simulink model "case9"  (R2024b)
settings: Solver=FixedStepAuto  StartTime=0  StopTime=1  FixedStep=1e-7  RelTol=1e-3
values from neighbouring files (symbols this model uses):
  SG_D_1_D = 0.01056    [IEEE9_case_parameters.m]    (also in case1_parameters.m; case2_parameters.m; case3_parameters.m; case4_parameters.m)
  SG_D_1_EnableSaturation = 0    [IEEE9_case_parameters.m]    (also in case1_parameters.m; case2_parameters.m; case3_parameters.m; case4_parameters.m)
  SG_D_1_f0 = 60    [IEEE9_case_parameters.m]    (also in case1_parameters.m; case2_parameters.m; case3_parameters.m; case4_parameters.m)
  SG_D_1_H = 7.5    [IEEE9_case_parameters.m]    (also in case1_parameters.m; case2_parameters.m; case3_parameters.m; case4_parameters.m)
  SG_D_1_K_A = 20    [IEEE9_case_parameters.m]    (also in case1_parameters.m; case2_parameters.m; case3_parameters.m; case4_parameters.m)
  SG_D_1_K_E = 1.000000e+1    (= 10)    [IEEE9_case_parameters.m]    (also in case1_parameters.m; case2_parameters.m; case3_parameters.m; case4_parameters.m)
  SG_D_1_K_F = 2.363    [IEEE9_case_parameters.m]    (also in case1_parameters.m; case2_parameters.m; case3_parameters.m; case4_parameters.m)
  SG_D_1_K_s = 0.5    [IEEE9_case_parameters.m]    (also in case1_parameters.m = 5; case2_parameters.m = 5; case3_parameters.m = 5; case4_parameters.m = 5)
  SG_D_1_R_a = 0.001088    [IEEE9_case_parameters.m]    (also in case1_parameters.m; case2_parameters.m; case3_parameters.m; case4_parameters.m)
  SG_D_1_S_A = 1    [IEEE9_case_parameters.m]    (also in case1_parameters.m; case2_parameters.m; case3_parameters.m; case4_parameters.m)
  SG_D_1_S_B = 0.103    [IEEE9_case_parameters.m]    (also in case1_parameters.m; case2_parameters.m; case3_parameters.m; case4_parameters.m)
  SG_D_1_S_N = 10.659857    [IEEE9_case_parameters.m]    (also in case1_parameters.m; case2_parameters.m; case3_parameters.m; case4_parameters.m)
  SG_D_1_SpeedPara = 200    [IEEE9_case_parameters.m]    (also in case1_parameters.m; case2_parameters.m; case3_parameters.m; case4_parameters.m)
  SG_D_1_T_0 = 0.720173    [IEEE9_case_parameters.m]    (also in case1_parameters.m = 0.755522; case2_parameters.m = 0.808931; case3_parameters.m = 0.869402; case4_parameters.m = 0.729316)
  SG_D_1_T_1 = 0.3    [IEEE9_case_parameters.m]    (also in case1_parameters.m; case2_parameters.m; case3_parameters.m; case4_parameters.m)
  SG_D_1_T_2 = 0.05    [IEEE9_case_parameters.m]    (also in case1_parameters.m; case2_parameters.m; case3_parameters.m; case4_parameters.m)
  SG_D_1_T_3 = 0.02    [IEEE9_case_parameters.m]    (also in case1_parameters.m; case2_parameters.m; case3_parameters.m; case4_parameters.m)
  SG_D_1_T_4 = 0.005    [IEEE9_case_parameters.m]    (also in case1_parameters.m; case2_parameters.m; case3_parameters.m; case4_parameters.m)
  SG_D_1_T_A = 0.02    [IEEE9_case_parameters.m]    (also in case1_parameters.m; case2_parameters.m; case3_parameters.m; case4_parameters.m)
  SG_D_1_T_dd = 8.000000e+0    (= 8)    [IEEE9_case_parameters.m]    (also in case1_parameters.m; case2_parameters.m; case3_parameters.m; case4_parameters.m)
  SG_D_1_T_ddd = 0.04    [IEEE9_case_parameters.m]    (also in case1_parameters.m; case2_parameters.m; case3_parameters.m; case4_parameters.m)
  SG_D_1_T_E = 0.314    [IEEE9_case_parameters.m]    (also in case1_parameters.m; case2_parameters.m; case3_parameters.m; case4_parameters.m)
  SG_D_1_T_F = 0.35    [IEEE9_case_parameters.m]    (also in case1_parameters.m; case2_parameters.m; case3_parameters.m; case4_parameters.m)
  SG_D_1_T_qd = 0.8    [IEEE9_case_parameters.m]    (also in case1_parameters.m; case2_parameters.m; case3_parameters.m; case4_parameters.m)
  SG_D_1_T_qdd = 0.02    [IEEE9_case_parameters.m]    (also in case1_parameters.m; case2_parameters.m; case3_parameters.m; case4_parameters.m)
  SG_D_1_T_speed = 0.1    [IEEE9_case_parameters.m]    (also in case1_parameters.m = 200; case2_parameters.m = 200; case3_parameters.m = 200; case4_parameters.m = 200)
  SG_D_1_T_w = 0.5    [IEEE9_case_parameters.m]    (also in case1_parameters.m; case2_parameters.m; case3_parameters.m; case4_parameters.m)
  SG_D_1_V_ref = 1.990276    [IEEE9_case_parameters.m]    (also in case1_parameters.m = 2.042296; case2_parameters.m = 2.051388; case3_parameters.m = 2.089584; case4_parameters.m = 2.01845)
  SG_D_1_w_ref = 376.991118    [IEEE9_case_parameters.m]    (also in case1_parameters.m; case2_parameters.m; case3_parameters.m; case4_parameters.m)
  SG_D_1_wb = 6.000000e+1    (= 60)    [IEEE9_case_parameters.m]    (also in case1_parameters.m; case2_parameters.m; case3_parameters.m; case4_parameters.m)
  SG_D_1_x_d = 1.9    [IEEE9_case_parameters.m]    (also in case1_parameters.m; case2_parameters.m; case3_parameters.m; case4_parameters.m)
  SG_D_1_x_dd = 0.302    [IEEE9_case_parameters.m]    (also in case1_parameters.m; case2_parameters.m; case3_parameters.m; case4_parameters.m)
  SG_D_1_x_ddd = 0.204    [IEEE9_case_parameters.m]    (also in case1_parameters.m; case2_parameters.m; case3_parameters.m; case4_parameters.m)
  SG_D_1_x_l = 0.05    [IEEE9_case_parameters.m]    (also in case1_parameters.m; case2_parameters.m; case3_parameters.m; case4_parameters.m)
  SG_D_1_x_q = 1.3    [IEEE9_case_parameters.m]    (also in case1_parameters.m; case2_parameters.m; case3_parameters.m; case4_parameters.m)
  SG_D_1_x_qd = 0.5    [IEEE9_case_parameters.m]    (also in case1_parameters.m; case2_parameters.m; case3_parameters.m; case4_parameters.m)
  SG_D_1_x_qdd = 0.3    [IEEE9_case_parameters.m]    (also in case1_parameters.m; case2_parameters.m; case3_parameters.m; case4_parameters.m)
  SG_D_2_D = 0.02    [IEEE9_case_parameters.m]    (also in case1_parameters.m; case2_parameters.m; case3_parameters.m; case4_parameters.m)
  SG_D_2_EnableSaturation = 0    [IEEE9_case_parameters.m]    (also in case1_parameters.m; case2_parameters.m; case3_parameters.m; case4_parameters.m)
  SG_D_2_f0 = 60    [IEEE9_case_parameters.m]    (also in case1_parameters.m; case2_parameters.m; case3_parameters.m; case4_parameters.m)
  SG_D_2_H = 8.000000e+0    (= 8)    [IEEE9_case_parameters.m]    (also in case1_parameters.m; case2_parameters.m; case3_parameters.m; case4_parameters.m)
  SG_D_2_K_A = 20    [IEEE9_case_parameters.m]    (also in case1_parameters.m; case2_parameters.m; case3_parameters.m; case4_parameters.m)
  SG_D_2_K_E = 1.000000e+1    (= 10)    [IEEE9_case_parameters.m]    (also in case1_parameters.m; case2_parameters.m; case3_parameters.m; case4_parameters.m)
  SG_D_2_K_F = 2.363    [IEEE9_case_parameters.m]    (also in case1_parameters.m; case2_parameters.m; case3_parameters.m; case4_parameters.m)
  SG_D_2_K_s = 0.5    [IEEE9_case_parameters.m]    (also in case1_parameters.m = 4; case2_parameters.m = 4; case3_parameters.m = 4; case4_parameters.m = 4)
  SG_D_2_R_a = 0.001088    [IEEE9_case_parameters.m]    (also in case1_parameters.m; case2_parameters.m; case3_parameters.m; case4_parameters.m)
  SG_D_2_S_A = 1    [IEEE9_case_parameters.m]    (also in case1_parameters.m; case2_parameters.m; case3_parameters.m; case4_parameters.m)
  SG_D_2_S_B = 0.103    [IEEE9_case_parameters.m]    (also in case1_parameters.m; case2_parameters.m; case3_parameters.m; case4_parameters.m)
  SG_D_2_S_N = 10.659857    [IEEE9_case_parameters.m]    (also in case1_parameters.m; case2_parameters.m; case3_parameters.m; case4_parameters.m)
  SG_D_2_SpeedPara = 200    [IEEE9_case_parameters.m]    (also in case1_parameters.m; case2_parameters.m; case3_parameters.m; case4_parameters.m)
  SG_D_2_T_0 = 1.632913    [IEEE9_case_parameters.m]    (also in case1_parameters.m = 1.632925; case2_parameters.m = 1.632915; case3_parameters.m = 1.632914; case4_parameters.m = 1.632927)
  SG_D_2_T_1 = 0.2    [IEEE9_case_parameters.m]    (also in case1_parameters.m; case2_parameters.m; case3_parameters.m; case4_parameters.m)
  SG_D_2_T_2 = 0.05    [IEEE9_case_parameters.m]    (also in case1_parameters.m; case2_parameters.m; case3_parameters.m; case4_parameters.m)
  SG_D_2_T_3 = 0.02    [IEEE9_case_parameters.m]    (also in case1_parameters.m; case2_parameters.m; case3_parameters.m; case4_parameters.m)
  SG_D_2_T_4 = 0.005    [IEEE9_case_parameters.m]    (also in case1_parameters.m; case2_parameters.m; case3_parameters.m; case4_parameters.m)
  SG_D_2_T_A = 0.02    [IEEE9_case_parameters.m]    (also in case1_parameters.m; case2_parameters.m; case3_parameters.m; case4_parameters.m)
  SG_D_2_T_dd = 7.9    [IEEE9_case_parameters.m]    (also in case1_parameters.m; case2_parameters.m; case3_parameters.m; case4_parameters.m)
  SG_D_2_T_ddd = 0.04    [IEEE9_case_parameters.m]    (also in case1_parameters.m; case2_parameters.m; case3_parameters.m; case4_parameters.m)
  SG_D_2_T_E = 0.314    [IEEE9_case_parameters.m]    (also in case1_parameters.m; case2_parameters.m; case3_parameters.m; case4_parameters.m)
  SG_D_2_T_F = 0.35    [IEEE9_case_parameters.m]    (also in case1_parameters.m; case2_parameters.m; case3_parameters.m; case4_parameters.m)
  SG_D_2_T_qd = 0.8    [IEEE9_case_parameters.m]    (also in case1_parameters.m; case2_parameters.m; case3_parameters.m; case4_parameters.m)
  SG_D_2_T_qdd = 0.015    [IEEE9_case_parameters.m]    (also in case1_parameters.m; case2_parameters.m; case3_parameters.m; case4_parameters.m)
  SG_D_2_T_speed = 0.1    [IEEE9_case_parameters.m]    (also in case1_parameters.m = 150; case2_parameters.m = 150; case3_parameters.m = 150; case4_parameters.m = 150)
  SG_D_2_T_w = 0.35    [IEEE9_case_parameters.m]    (also in case1_parameters.m; case2_parameters.m; case3_parameters.m; case4_parameters.m)
  SG_D_2_V_ref = 2.58547    [IEEE9_case_parameters.m]    (also in case1_parameters.m = 2.597896; case2_parameters.m = 2.587136; case3_parameters.m = 2.586042; case4_parameters.m = 2.599679)
  SG_D_2_w_ref = 376.991118    [IEEE9_case_parameters.m]    (also in case1_parameters.m; case2_parameters.m; case3_parameters.m; case4_parameters.m)
  SG_D_2_wb = 6.000000e+1    (= 60)    [IEEE9_case_parameters.m]    (also in case1_parameters.m; case2_parameters.m; case3_parameters.m; case4_parameters.m)
  SG_D_2_x_d = 1.8    [IEEE9_case_parameters.m]    (also in case1_parameters.m; case2_parameters.m; case3_parameters.m; case4_parameters.m)
  SG_D_2_x_dd = 0.302    [IEEE9_case_parameters.m]    (also in case1_parameters.m; case2_parameters.m; case3_parameters.m; case4_parameters.m)
  SG_D_2_x_ddd = 0.204    [IEEE9_case_parameters.m]    (also in case1_parameters.m; case2_parameters.m; case3_parameters.m; case4_parameters.m)
  SG_D_2_x_l = 0.05    [IEEE9_case_parameters.m]    (also in case1_parameters.m; case2_parameters.m; case3_parameters.m; case4_parameters.m)
  SG_D_2_x_q = 1.25    [IEEE9_case_parameters.m]    (also in case1_parameters.m; case2_parameters.m; case3_parameters.m; case4_parameters.m)
  SG_D_2_x_qd = 0.5    [IEEE9_case_parameters.m]    (also in case1_parameters.m; case2_parameters.m; case3_parameters.m; case4_parameters.m)
  SG_D_2_x_qdd = 0.3    [IEEE9_case_parameters.m]    (also in case1_parameters.m; case2_parameters.m; case3_parameters.m; case4_parameters.m)
  SG_D_3_D = 0.02    [IEEE9_case_parameters.m]    (also in case1_parameters.m; case2_parameters.m; case3_parameters.m; case4_parameters.m)
  SG_D_3_EnableSaturation = 0    [IEEE9_case_parameters.m]    (also in case1_parameters.m; case2_parameters.m; case3_parameters.m; case4_parameters.m)
  SG_D_3_f0 = 60    [IEEE9_case_parameters.m]    (also in case1_parameters.m; case2_parameters.m; case3_parameters.m; case4_parameters.m)
  SG_D_3_H = 7.7    [IEEE9_case_parameters.m]    (also in case1_parameters.m; case2_parameters.m; case3_parameters.m; case4_parameters.m)
  SG_D_3_K_A = 20    [IEEE9_case_parameters.m]    (also in case1_parameters.m; case2_parameters.m; case3_parameters.m; case4_parameters.m)
  SG_D_3_K_E = 1.000000e+1    (= 10)    [IEEE9_case_parameters.m]    (also in case1_parameters.m; case2_parameters.m; case3_parameters.m; case4_parameters.m)
  SG_D_3_K_F = 2.363    [IEEE9_case_parameters.m]    (also in case1_parameters.m; case2_parameters.m; case3_parameters.m; case4_parameters.m)
  SG_D_3_K_s = 0.2    [IEEE9_case_parameters.m]    (also in case1_parameters.m = 2; case2_parameters.m = 2; case3_parameters.m = 2; case4_parameters.m = 2)
  SG_D_3_R_a = 0.001088    [IEEE9_case_parameters.m]    (also in case1_parameters.m; case2_parameters.m; case3_parameters.m; case4_parameters.m)
  SG_D_3_S_A = 1    [IEEE9_case_parameters.m]    (also in case1_parameters.m; case2_parameters.m; case3_parameters.m; case4_parameters.m)
  SG_D_3_S_B = 0.103    [IEEE9_case_parameters.m]    (also in case1_parameters.m; case2_parameters.m; case3_parameters.m; case4_parameters.m)
  SG_D_3_S_N = 10.659857    [IEEE9_case_parameters.m]    (also in case1_parameters.m; case2_parameters.m; case3_parameters.m; case4_parameters.m)
  SG_D_3_SpeedPara = 200    [IEEE9_case_parameters.m]    (also in case1_parameters.m; case2_parameters.m; case3_parameters.m; case4_parameters.m)
  SG_D_3_T_0 = 0.850788    [IEEE9_case_parameters.m]    (also in case1_parameters.m = 0.850786; case2_parameters.m = 0.850787; case3_parameters.m; case4_parameters.m = 0.850786)
  SG_D_3_T_1 = 0.2    [IEEE9_case_parameters.m]    (also in case1_parameters.m; case2_parameters.m; case3_parameters.m; case4_parameters.m)
  SG_D_3_T_2 = 0.05    [IEEE9_case_parameters.m]    (also in case1_parameters.m; case2_parameters.m; case3_parameters.m; case4_parameters.m)
  SG_D_3_T_3 = 0.02    [IEEE9_case_parameters.m]    (also in case1_parameters.m; case2_parameters.m; case3_parameters.m; case4_parameters.m)
  SG_D_3_T_4 = 0.005    [IEEE9_case_parameters.m]    (also in case1_parameters.m; case2_parameters.m; case3_parameters.m; case4_parameters.m)
  SG_D_3_T_A = 0.02    [IEEE9_case_parameters.m]    (also in case1_parameters.m; case2_parameters.m; case3_parameters.m; case4_parameters.m)
  SG_D_3_T_dd = 8.1    [IEEE9_case_parameters.m]    (also in case1_parameters.m; case2_parameters.m; case3_parameters.m; case4_parameters.m)
  SG_D_3_T_ddd = 0.04    [IEEE9_case_parameters.m]    (also in case1_parameters.m; case2_parameters.m; case3_parameters.m; case4_parameters.m)
  SG_D_3_T_E = 0.314    [IEEE9_case_parameters.m]    (also in case1_parameters.m; case2_parameters.m; case3_parameters.m; case4_parameters.m)
  SG_D_3_T_F = 0.35    [IEEE9_case_parameters.m]    (also in case1_parameters.m; case2_parameters.m; case3_parameters.m; case4_parameters.m)
  SG_D_3_T_qd = 0.8    [IEEE9_case_parameters.m]    (also in case1_parameters.m; case2_parameters.m; case3_parameters.m; case4_parameters.m)
  SG_D_3_T_qdd = 0.015    [IEEE9_case_parameters.m]    (also in case1_parameters.m; case2_parameters.m; case3_parameters.m; case4_parameters.m)
  SG_D_3_T_speed = 0.1    [IEEE9_case_parameters.m]    (also in case1_parameters.m = 180; case2_parameters.m = 180; case3_parameters.m = 180; case4_parameters.m = 180)
  SG_D_3_T_w = 0.4    [IEEE9_case_parameters.m]    (also in case1_parameters.m; case2_parameters.m; case3_parameters.m; case4_parameters.m)
  SG_D_3_V_ref = 1.892727    [IEEE9_case_parameters.m]    (also in case1_parameters.m = 1.906439; case2_parameters.m = 1.895535; case3_parameters.m = 1.892105; case4_parameters.m = 1.906598)
  SG_D_3_w_ref = 376.991118    [IEEE9_case_parameters.m]    (also in case1_parameters.m; case2_parameters.m; case3_parameters.m; case4_parameters.m)
  SG_D_3_wb = 6.000000e+1    (= 60)    [IEEE9_case_parameters.m]    (also in case1_parameters.m; case2_parameters.m; case3_parameters.m; case4_parameters.m)
  SG_D_3_x_d = 1.85    [IEEE9_case_parameters.m]    (also in case1_parameters.m; case2_parameters.m; case3_parameters.m; case4_parameters.m)
  SG_D_3_x_dd = 0.302    [IEEE9_case_parameters.m]    (also in case1_parameters.m; case2_parameters.m; case3_parameters.m; case4_parameters.m)
  SG_D_3_x_ddd = 0.204    [IEEE9_case_parameters.m]    (also in case1_parameters.m; case2_parameters.m; case3_parameters.m; case4_parameters.m)
  SG_D_3_x_l = 0.05    [IEEE9_case_parameters.m]    (also in case1_parameters.m; case2_parameters.m; case3_parameters.m; case4_parameters.m)
  SG_D_3_x_q = 1.2    [IEEE9_case_parameters.m]    (also in case1_parameters.m; case2_parameters.m; case3_parameters.m; case4_parameters.m)
  SG_D_3_x_qd = 0.5    [IEEE9_case_parameters.m]    (also in case1_parameters.m; case2_parameters.m; case3_parameters.m; case4_parameters.m)
  SG_D_3_x_qdd = 0.3    [IEEE9_case_parameters.m]    (also in case1_parameters.m; case2_parameters.m; case3_parameters.m; case4_parameters.m)
(part 2 of 12)

== system case9/AC_1/d_id_line_8_9_block ==
  note: d_id_line_8_9 in case9
      | $376.991118430775\,\mathrm{iq}_{\mathrm{line},8,9}-79.079547273782\,\mathrm{id}_{\mathrm{line},8,9}+2308.03849601368\,\mathrm{vd}_{\mathrm{bus},8}-2308.03849601368\,\mathrm{vd}_{\mathrm{bus},9}$
      | Automatically generated on 2025-10-31 19:35:46 .
  State_id_line_8_9_7f57b : Inport
  State_iq_line_8_9_a0851 : Inport  Port=2
  State_vd_bus_8_2850b : Inport  Port=3
  State_vd_bus_9_05d0b : Inport  Port=4
  Add_7d5a3 : Sum
  Add_dee88 : Sum
  Constant_-79.079547273782_7223d : Constant  Value=-79.079547273782
  Constant_2308.03849601368_486f2 : Constant  Value=2308.03849601368
  Constant_2308.03849601368_a27ee : Constant  Value=2308.03849601368
  Constant_376.991118430775_3d7fd : Constant  Value=376.991118430775
  Product_07161 : Product
  Product_cf3c9 : Product
  Product_d47ae : Product
  Product_f756a : Product
  Subtract_736c3 : Sum  Inputs=+-
  Blockout_d_id_line_8_9_34a3f : Outport
  wires:
  Constant_-79.079547273782_7223d/1 -> Product_d47ae/1
  Product_f756a/1 -> Add_7d5a3/2
  State_id_line_8_9_7f57b/1 -> Product_d47ae/2
  Constant_376.991118430775_3d7fd/1 -> Product_f756a/1
  State_iq_line_8_9_a0851/1 -> Product_f756a/2
  Product_d47ae/1 -> Add_7d5a3/1
  Constant_2308.03849601368_486f2/1 -> Product_07161/1
  State_vd_bus_8_2850b/1 -> Product_07161/2
  Add_7d5a3/1 -> Add_dee88/1
  Product_07161/1 -> Add_dee88/2
  Constant_2308.03849601368_a27ee/1 -> Product_cf3c9/1
  State_vd_bus_9_05d0b/1 -> Product_cf3c9/2
  Add_dee88/1 -> Subtract_736c3/1
  Product_cf3c9/1 -> Subtract_736c3/2
  Subtract_736c3/1 -> Blockout_d_id_line_8_9_34a3f/1

== system case9/AC_1/d_id_line_9_4_block ==
  note: d_id_line_9_4 in case9
      | $376.991118430775\,\mathrm{iq}_{\mathrm{line},9,4}-46.8081143789666\,\mathrm{id}_{\mathrm{line},9,4}-4371.69644539061\,\mathrm{vd}_{\mathrm{bus},4}+4371.69644539061\,\mathrm{vd}_{\mathrm{bus},9}$
      | Automatically generated on 2025-10-31 19:35:47 .
  State_id_line_9_4_2f88c : Inport
  State_iq_line_9_4_5e3d8 : Inport  Port=2
  State_vd_bus_4_6d2a8 : Inport  Port=3
  State_vd_bus_9_2d37e : Inport  Port=4
  Add_5ea3d : Sum
  Add_7fd3a : Sum
  Constant_-46.8081143789666_5ee22 : Constant  Value=-46.8081143789666
  Constant_376.991118430775_a2f3b : Constant  Value=376.991118430775
  Constant_4371.69644539061_67045 : Constant  Value=4371.69644539061
  Constant_4371.69644539061_93ce0 : Constant  Value=4371.69644539061
  Product_23b32 : Product
  Product_5d2fa : Product
  Product_c4883 : Product
  Product_f07a4 : Product
  Subtract_26f71 : Sum  Inputs=+-
  Blockout_d_id_line_9_4_009d8 : Outport
  wires:
  Constant_-46.8081143789666_5ee22/1 -> Product_c4883/1
  Product_23b32/1 -> Add_5ea3d/2
  State_id_line_9_4_2f88c/1 -> Product_c4883/2
  Constant_376.991118430775_a2f3b/1 -> Product_23b32/1
  Product_c4883/1 -> Add_5ea3d/1
  State_iq_line_9_4_5e3d8/1 -> Product_23b32/2
  Constant_4371.69644539061_67045/1 -> Product_f07a4/1
  State_vd_bus_4_6d2a8/1 -> Product_f07a4/2
  Add_5ea3d/1 -> Subtract_26f71/1
  Product_f07a4/1 -> Subtract_26f71/2
  Constant_4371.69644539061_93ce0/1 -> Product_5d2fa/1
  Subtract_26f71/1 -> Add_7fd3a/1
  State_vd_bus_9_2d37e/1 -> Product_5d2fa/2
  Product_5d2fa/1 -> Add_7fd3a/2
  Add_7fd3a/1 -> Blockout_d_id_line_9_4_009d8/1

== system case9/AC_1/d_id_load_5_block ==
  note: d_id_load_5 in case9
      | $376.991118430775\,\mathrm{iq}_{\mathrm{load},5}-1271.35173163011\,\mathrm{id}_{\mathrm{load},5}+1369.24920855552\,\mathrm{vd}_{\mathrm{bus},5}$
      | Automatically generated on 2025-10-31 19:35:37 .
  State_id_load_5_0cf96 : Inport
  State_iq_load_5_0d2e0 : Inport  Port=2
  State_vd_bus_5_6d5a2 : Inport  Port=3
  Add_3aace : Sum
  Add_6ece1 : Sum
  Constant_-1271.35173163011_4a864 : Constant  Value=-1271.35173163011
  Constant_1369.24920855552_9b5a8 : Constant  Value=1369.24920855552
  Constant_376.991118430775_69578 : Constant  Value=376.991118430775
  Product_78272 : Product
  Product_da222 : Product
  Product_dfef5 : Product
  Blockout_d_id_load_5_39313 : Outport
  wires:
  Constant_-1271.35173163011_4a864/1 -> Product_78272/1
  Product_dfef5/1 -> Add_6ece1/2
  State_id_load_5_0cf96/1 -> Product_78272/2
  Constant_376.991118430775_69578/1 -> Product_dfef5/1
  Product_da222/1 -> Add_3aace/2
  State_iq_load_5_0d2e0/1 -> Product_dfef5/2
  Product_78272/1 -> Add_6ece1/1
  Constant_1369.24920855552_9b5a8/1 -> Product_da222/1
  State_vd_bus_5_6d5a2/1 -> Product_da222/2
  Add_6ece1/1 -> Add_3aace/1
  Add_3aace/1 -> Blockout_d_id_load_5_39313/1

== system case9/AC_1/d_id_load_7_block ==
  note: d_id_load_7 in case9
      | $376.991118430775\,\mathrm{iq}_{\mathrm{load},7}-1210.81117316871\,\mathrm{id}_{\mathrm{load},7}+1430.28886940914\,\mathrm{vd}_{\mathrm{bus},7}$
      | Automatically generated on 2025-10-31 19:35:38 .
  State_id_load_7_475ab : Inport
  State_iq_load_7_faf72 : Inport  Port=2
  State_vd_bus_7_54001 : Inport  Port=3
  Add_78a86 : Sum
  Add_d7d34 : Sum
  Constant_-1210.81117316871_adc5d : Constant  Value=-1210.81117316871
  Constant_1430.28886940914_d6361 : Constant  Value=1430.28886940914
  Constant_376.991118430775_fd455 : Constant  Value=376.991118430775
  Product_c0859 : Product
  Product_ea5b8 : Product
  Product_fa99e : Product
  Blockout_d_id_load_7_24cac : Outport
  wires:
  Constant_-1210.81117316871_adc5d/1 -> Product_fa99e/1
  Product_c0859/1 -> Add_78a86/2
  State_id_load_7_475ab/1 -> Product_fa99e/2
  Constant_376.991118430775_fd455/1 -> Product_c0859/1
  Product_fa99e/1 -> Add_78a86/1
  State_iq_load_7_faf72/1 -> Product_c0859/2
  Constant_1430.28886940914_d6361/1 -> Product_ea5b8/1
  State_vd_bus_7_54001/1 -> Product_ea5b8/2
  Add_78a86/1 -> Add_d7d34/1
  Product_ea5b8/1 -> Add_d7d34/2
  Add_d7d34/1 -> Blockout_d_id_load_7_24cac/1

== system case9/AC_1/d_id_load_9_block ==
  note: d_id_load_9 in case9
      | $376.991118430775\,\mathrm{iq}_{\mathrm{load},9}-1059.45977647\,\mathrm{id}_{\mathrm{load},9}+1700.21710984812\,\mathrm{vd}_{\mathrm{bus},9}$
      | Automatically generated on 2025-10-31 19:35:39 .
  State_id_load_9_9c654 : Inport
  State_iq_load_9_9f0e2 : Inport  Port=2
  State_vd_bus_9_61c11 : Inport  Port=3
  Add_3c334 : Sum
  Add_4cb1c : Sum
  Constant_-1059.45977647_80d06 : Constant  Value=-1059.45977647
  Constant_1700.21710984812_ffb11 : Constant  Value=1700.21710984812
  Constant_376.991118430775_49f56 : Constant  Value=376.991118430775
  Product_15e95 : Product
  Product_2c0b1 : Product
  Product_f7556 : Product
  Blockout_d_id_load_9_7efdf : Outport
  wires:
  Constant_-1059.45977647_80d06/1 -> Product_15e95/1
  Product_2c0b1/1 -> Add_3c334/2
  State_id_load_9_9c654/1 -> Product_15e95/2
  Constant_376.991118430775_49f56/1 -> Product_2c0b1/1
  Product_15e95/1 -> Add_3c334/1
  State_iq_load_9_9f0e2/1 -> Product_2c0b1/2
  Constant_1700.21710984812_ffb11/1 -> Product_f7556/1
  State_vd_bus_9_61c11/1 -> Product_f7556/2
  Add_3c334/1 -> Add_4cb1c/1
  Product_f7556/1 -> Add_4cb1c/2
  Add_4cb1c/1 -> Blockout_d_id_load_9_7efdf/1

== system case9/AC_1/d_iq_line_1_4_block ==
  note: d_iq_line_1_4 in case9
      | $6451.28815726045\,\mathrm{vq}_{\mathrm{bus},1}-376.991118430775\,\mathrm{id}_{\mathrm{line},1,4}-6451.28815726045\,\mathrm{vq}_{\mathrm{bus},4}$
      | Automatically generated on 2025-10-31 19:35:40 .
  State_id_line_1_4_4a24e : Inport
  State_vq_bus_1_3337a : Inport  Port=2
  State_vq_bus_4_a6b34 : Inport  Port=3
  Add_6db9b : Sum
  Constant_-376.991118430775_70d78 : Constant  Value=-376.991118430775
  Constant_6451.28815726045_2aa38 : Constant  Value=6451.28815726045
  Constant_6451.28815726045_82ff4 : Constant  Value=6451.28815726045
  Product_6c42f : Product
  Product_b527a : Product
  Product_fcdd1 : Product
  Subtract_113de : Sum  Inputs=+-
  Blockout_d_iq_line_1_4_3376e : Outport
  wires:
  Constant_-376.991118430775_70d78/1 -> Product_b527a/1
  Product_fcdd1/1 -> Add_6db9b/2
  State_id_line_1_4_4a24e/1 -> Product_b527a/2
  Constant_6451.28815726045_82ff4/1 -> Product_fcdd1/1
  Product_b527a/1 -> Add_6db9b/1
  Subtract_113de/1 -> Blockout_d_iq_line_1_4_3376e/1
  State_vq_bus_1_3337a/1 -> Product_fcdd1/2
  Constant_6451.28815726045_2aa38/1 -> Product_6c42f/1
  State_vq_bus_4_a6b34/1 -> Product_6c42f/2
  Add_6db9b/1 -> Subtract_113de/1
  Product_6c42f/1 -> Subtract_113de/2

== system case9/AC_1/d_iq_line_3_6_block ==
  note: d_iq_line_3_6 in case9
      | $6341.19791566897\,\mathrm{vq}_{\mathrm{bus},3}-376.991118430775\,\mathrm{id}_{\mathrm{line},3,6}-6341.19791566897\,\mathrm{vq}_{\mathrm{bus},6}$
      | Automatically generated on 2025-10-31 19:35:43 .
  State_id_line_3_6_aaf98 : Inport
  State_vq_bus_3_d110b : Inport  Port=2
  State_vq_bus_6_cc5e9 : Inport  Port=3
  Add_271bd : Sum
  Constant_-376.991118430775_89aa7 : Constant  Value=-376.991118430775
  Constant_6341.19791566897_20e3c : Constant  Value=6341.19791566897
  Constant_6341.19791566897_be9af : Constant  Value=6341.19791566897
  Product_900cb : Product
  Product_e38f3 : Product
  Product_e9343 : Product
  Subtract_02134 : Sum  Inputs=+-
  Blockout_d_iq_line_3_6_fff78 : Outport
  wires:
  Constant_-376.991118430775_89aa7/1 -> Product_e38f3/1
  Product_e9343/1 -> Add_271bd/2
  State_id_line_3_6_aaf98/1 -> Product_e38f3/2
  Constant_6341.19791566897_20e3c/1 -> Product_e9343/1
  Product_e38f3/1 -> Add_271bd/1
  State_vq_bus_3_d110b/1 -> Product_e9343/2
  Constant_6341.19791566897_be9af/1 -> Product_900cb/1
  State_vq_bus_6_cc5e9/1 -> Product_900cb/2
  Add_271bd/1 -> Subtract_02134/1
  Product_900cb/1 -> Subtract_02134/2
  Subtract_02134/1 -> Blockout_d_iq_line_3_6_fff78/1

== system case9/AC_1/d_iq_line_4_5_block ==
  note: d_iq_line_4_5 in case9
      | $4039.06736802393\,\mathrm{vq}_{\mathrm{bus},4}-73.5192666060942\,\mathrm{iq}_{\mathrm{line},4,5}-376.991118430775\,\mathrm{id}_{\mathrm{line},4,5}-4039.06736802393\,\mathrm{vq}_{\mathrm{bus},5}$
      | Automatically generated on 2025-10-31 19:35:41 .
  State_id_line_4_5_16899 : Inport
  State_iq_line_4_5_7ec19 : Inport  Port=2
  State_vq_bus_4_25c97 : Inport  Port=3
  State_vq_bus_5_9266e : Inport  Port=4
  Add_c2a52 : Sum
  Constant_-376.991118430775_7560b : Constant  Value=-376.991118430775
  Constant_4039.06736802393_a496b : Constant  Value=4039.06736802393
  Constant_4039.06736802393_bc54f : Constant  Value=4039.06736802393
  Constant_73.5192666060942_9a8aa : Constant  Value=73.5192666060942
  Product_06954 : Product
  Product_7bca2 : Product
  Product_956c9 : Product
  Product_c538f : Product
  Subtract_1ae29 : Sum  Inputs=+-
  Subtract_47e43 : Sum  Inputs=+-
  Blockout_d_iq_line_4_5_383ee : Outport
  wires:
  Constant_-376.991118430775_7560b/1 -> Product_c538f/1
  Constant_73.5192666060942_9a8aa/1 -> Product_956c9/1
  State_id_line_4_5_16899/1 -> Product_c538f/2
  State_iq_line_4_5_7ec19/1 -> Product_956c9/2
  Product_c538f/1 -> Subtract_1ae29/1
  Constant_4039.06736802393_bc54f/1 -> Product_7bca2/1
  Product_956c9/1 -> Subtract_1ae29/2
  State_vq_bus_4_25c97/1 -> Product_7bca2/2
  Subtract_1ae29/1 -> Add_c2a52/1
  Product_7bca2/1 -> Add_c2a52/2
  Constant_4039.06736802393_a496b/1 -> Product_06954/1
  State_vq_bus_5_9266e/1 -> Product_06954/2
  Add_c2a52/1 -> Subtract_47e43/1
  Product_06954/1 -> Subtract_47e43/2
  Subtract_47e43/1 -> Blockout_d_iq_line_4_5_383ee/1

== system case9/AC_1/d_iq_line_5_6_block ==
  note: d_iq_line_5_6 in case9
      | $2185.8482226953\,\mathrm{vq}_{\mathrm{bus},5}-91.2758230389848\,\mathrm{iq}_{\mathrm{line},5,6}-376.991118430775\,\mathrm{id}_{\mathrm{line},5,6}-2185.8482226953\,\mathrm{vq}_{\mathrm{bus},6}$
      | Automatically generated on 2025-10-31 19:35:42 .
  State_id_line_5_6_afd48 : Inport
  State_iq_line_5_6_efdcc : Inport  Port=2
  State_vq_bus_5_b416f : Inport  Port=3
  State_vq_bus_6_d5e8e : Inport  Port=4
  Add_2264d : Sum
  Constant_-376.991118430775_0d3a9 : Constant  Value=-376.991118430775
  Constant_2185.8482226953_84ed3 : Constant  Value=2185.8482226953
  Constant_2185.8482226953_fd645 : Constant  Value=2185.8482226953
  Constant_91.2758230389848_739b5 : Constant  Value=91.2758230389848
  Product_54809 : Product
  Product_7a7b1 : Product
  Product_bd2b0 : Product
  Product_fb77b : Product
  Subtract_2ef38 : Sum  Inputs=+-
  Subtract_f2d37 : Sum  Inputs=+-
  Blockout_d_iq_line_5_6_5c2d3 : Outport
  wires:
  Constant_-376.991118430775_0d3a9/1 -> Product_7a7b1/1
  Constant_91.2758230389848_739b5/1 -> Product_bd2b0/1
  Subtract_2ef38/1 -> Blockout_d_iq_line_5_6_5c2d3/1
  State_id_line_5_6_afd48/1 -> Product_7a7b1/2
  State_iq_line_5_6_efdcc/1 -> Product_bd2b0/2
  Product_7a7b1/1 -> Subtract_f2d37/1
  Constant_2185.8482226953_84ed3/1 -> Product_fb77b/1
  Product_bd2b0/1 -> Subtract_f2d37/2
  Product_54809/1 -> Subtract_2ef38/2
  State_vq_bus_5_b416f/1 -> Product_fb77b/2
  Subtract_f2d37/1 -> Add_2264d/1
  Product_fb77b/1 -> Add_2264d/2
  Constant_2185.8482226953_fd645/1 -> Product_54809/1
  State_vq_bus_6_d5e8e/1 -> Product_54809/2
  Add_2264d/1 -> Subtract_2ef38/1

== system case9/AC_1/d_iq_line_6_7_block ==
  note: d_iq_line_6_7 in case9
      | $3686.4503755774\,\mathrm{vq}_{\mathrm{bus},6}-46.9706425538935\,\mathrm{iq}_{\mathrm{line},6,7}-376.991118430775\,\mathrm{id}_{\mathrm{line},6,7}-3686.4503755774\,\mathrm{vq}_{\mathrm{bus},7}$
      | Automatically generated on 2025-10-31 19:35:44 .
  State_id_line_6_7_6b997 : Inport
  State_iq_line_6_7_97013 : Inport  Port=2
  State_vq_bus_6_61006 : Inport  Port=3
  State_vq_bus_7_29567 : Inport  Port=4
  Add_ce773 : Sum
  Constant_-376.991118430775_9d153 : Constant  Value=-376.991118430775
  Constant_3686.4503755774_1893c : Constant  Value=3686.4503755774
  Constant_3686.4503755774_48d88 : Constant  Value=3686.4503755774
  Constant_46.9706425538935_c073d : Constant  Value=46.9706425538935
  Product_36a0b : Product
  Product_aef2d : Product
  Product_e57e7 : Product
  Product_f7d4b : Product
  Subtract_95771 : Sum  Inputs=+-
  Subtract_b4a81 : Sum  Inputs=+-
  Blockout_d_iq_line_6_7_15ad5 : Outport
  wires:
  Constant_-376.991118430775_9d153/1 -> Product_aef2d/1
  Constant_46.9706425538935_c073d/1 -> Product_e57e7/1
  State_id_line_6_7_6b997/1 -> Product_aef2d/2
  State_iq_line_6_7_97013/1 -> Product_e57e7/2
  Product_aef2d/1 -> Subtract_95771/1
  Constant_3686.4503755774_48d88/1 -> Product_f7d4b/1
  Product_e57e7/1 -> Subtract_95771/2
  State_vq_bus_6_61006/1 -> Product_f7d4b/2
  Subtract_95771/1 -> Add_ce773/1
  Product_f7d4b/1 -> Add_ce773/2
  Constant_3686.4503755774_1893c/1 -> Product_36a0b/1
  State_vq_bus_7_29567/1 -> Product_36a0b/2
  Add_ce773/1 -> Subtract_b4a81/1
  Product_36a0b/1 -> Subtract_b4a81/2
  Subtract_b4a81/1 -> Blockout_d_iq_line_6_7_15ad5/1

== system case9/AC_1/d_iq_line_7_8_block ==
  note: d_iq_line_7_8 in case9
      | $5161.03052580836\,\mathrm{vq}_{\mathrm{bus},7}-46.9706425538935\,\mathrm{iq}_{\mathrm{line},7,8}-376.991118430775\,\mathrm{id}_{\mathrm{line},7,8}-5161.03052580836\,\mathrm{vq}_{\mathrm{bus},8}$
      | Automatically generated on 2025-10-31 19:35:45 .
  State_id_line_7_8_d8e71 : Inport
  State_iq_line_7_8_1f96c : Inport  Port=2
  State_vq_bus_7_ddff2 : Inport  Port=3
  State_vq_bus_8_84832 : Inport  Port=4
  Add_d3133 : Sum
  Constant_-376.991118430775_f6390 : Constant  Value=-376.991118430775
  Constant_46.9706425538935_10800 : Constant  Value=46.9706425538935
  Constant_5161.03052580836_81b4f : Constant  Value=5161.03052580836
  Constant_5161.03052580836_a8f17 : Constant  Value=5161.03052580836
  Product_4753d : Product
  Product_73ab9 : Product
  Product_a1d16 : Product
  Product_e13d7 : Product
  Subtract_933c0 : Sum  Inputs=+-
  Subtract_e7f7e : Sum  Inputs=+-
  Blockout_d_iq_line_7_8_fd98e : Outport
  wires:
  Constant_-376.991118430775_f6390/1 -> Product_73ab9/1
  Constant_46.9706425538935_10800/1 -> Product_a1d16/1
  State_id_line_7_8_d8e71/1 -> Product_73ab9/2
  State_iq_line_7_8_1f96c/1 -> Product_a1d16/2
  Product_73ab9/1 -> Subtract_e7f7e/1
  Constant_5161.03052580836_a8f17/1 -> Product_4753d/1
  Product_a1d16/1 -> Subtract_e7f7e/2
  State_vq_bus_7_ddff2/1 -> Product_4753d/2
  Subtract_e7f7e/1 -> Add_d3133/1
  Product_4753d/1 -> Add_d3133/2
  Constant_5161.03052580836_81b4f/1 -> Product_e13d7/1
  State_vq_bus_8_84832/1 -> Product_e13d7/2
  Add_d3133/1 -> Subtract_933c0/1
  Product_e13d7/1 -> Subtract_933c0/2
  Subtract_933c0/1 -> Blockout_d_iq_line_7_8_fd98e/1

== system case9/AC_1/d_iq_line_8_2_block ==
  note: d_iq_line_8_2 in case9
      | $5945.50716573123\,\mathrm{vq}_{\mathrm{bus},8}-5945.50716573123\,\mathrm{vq}_{\mathrm{bus},2}-376.991118430775\,\mathrm{id}_{\mathrm{line},8,2}$
      | Automatically generated on 2025-10-31 19:35:45 .
  State_id_line_8_2_3b696 : Inport
  State_vq_bus_2_3fe0d : Inport  Port=2
  State_vq_bus_8_f943e : Inport  Port=3
  Add_1fa4b : Sum
  Constant_-376.991118430775_f5f9b : Constant  Value=-376.991118430775
  Constant_5945.50716573123_3ac16 : Constant  Value=5945.50716573123
  Constant_5945.50716573123_5db4d : Constant  Value=5945.50716573123
  Product_0c260 : Product
  Product_9bd1f : Product
  Product_a3333 : Product
  Subtract_22f9e : Sum  Inputs=+-
  Blockout_d_iq_line_8_2_ea60e : Outport
  wires:
  Constant_-376.991118430775_f5f9b/1 -> Product_9bd1f/1
  Product_0c260/1 -> Subtract_22f9e/2
  State_id_line_8_2_3b696/1 -> Product_9bd1f/2
  Constant_5945.50716573123_5db4d/1 -> Product_0c260/1
  Product_9bd1f/1 -> Subtract_22f9e/1
  State_vq_bus_2_3fe0d/1 -> Product_0c260/2
  Constant_5945.50716573123_3ac16/1 -> Product_a3333/1
  State_vq_bus_8_f943e/1 -> Product_a3333/2
  Subtract_22f9e/1 -> Add_1fa4b/1
  Product_a3333/1 -> Add_1fa4b/2
  Add_1fa4b/1 -> Blockout_d_iq_line_8_2_ea60e/1

== system case9/AC_1/d_iq_line_8_9_block ==
  note: d_iq_line_8_9 in case9
      | $2308.03849601368\,\mathrm{vq}_{\mathrm{bus},8}-79.079547273782\,\mathrm{iq}_{\mathrm{line},8,9}-376.991118430775\,\mathrm{id}_{\mathrm{line},8,9}-2308.03849601368\,\mathrm{vq}_{\mathrm{bus},9}$
      | Automatically generated on 2025-10-31 19:35:46 .
  State_id_line_8_9_c7584 : Inport
  State_iq_line_8_9_9dd27 : Inport  Port=2
  State_vq_bus_8_1c77b : Inport  Port=3
  State_vq_bus_9_c542c : Inport  Port=4
  Add_42656 : Sum
  Constant_-376.991118430775_bec13 : Constant  Value=-376.991118430775
  Constant_2308.03849601368_13c21 : Constant  Value=2308.03849601368
  Constant_2308.03849601368_17d42 : Constant  Value=2308.03849601368
  Constant_79.079547273782_9543b : Constant  Value=79.079547273782
  Product_08b87 : Product
  Product_24ad4 : Product
  Product_47dc7 : Product
  Product_a7821 : Product
  Subtract_3c3e0 : Sum  Inputs=+-
  Subtract_b8ab7 : Sum  Inputs=+-
  Blockout_d_iq_line_8_9_3c3a9 : Outport
  wires:
  Constant_-376.991118430775_bec13/1 -> Product_47dc7/1
  Constant_79.079547273782_9543b/1 -> Product_24ad4/1
  State_id_line_8_9_c7584/1 -> Product_47dc7/2
  State_iq_line_8_9_9dd27/1 -> Product_24ad4/2
  Product_47dc7/1 -> Subtract_b8ab7/1
  Constant_2308.03849601368_17d42/1 -> Product_a7821/1
  Product_24ad4/1 -> Subtract_b8ab7/2
  State_vq_bus_8_1c77b/1 -> Product_a7821/2
  Subtract_b8ab7/1 -> Add_42656/1
  Product_a7821/1 -> Add_42656/2
  Constant_2308.03849601368_13c21/1 -> Product_08b87/1
  Add_42656/1 -> Subtract_3c3e0/1
  State_vq_bus_9_c542c/1 -> Product_08b87/2
  Product_08b87/1 -> Subtract_3c3e0/2
  Subtract_3c3e0/1 -> Blockout_d_iq_line_8_9_3c3a9/1

== system case9/AC_1/d_iq_line_9_4_block ==
  note: d_iq_line_9_4 in case9
      | $4371.69644539061\,\mathrm{vq}_{\mathrm{bus},9}-46.8081143789666\,\mathrm{iq}_{\mathrm{line},9,4}-4371.69644539061\,\mathrm{vq}_{\mathrm{bus},4}-376.991118430775\,\mathrm{id}_{\mathrm{line},9,4}$
      | Automatically generated on 2025-10-31 19:35:47 .
  State_id_line_9_4_c69ca : Inport
  State_iq_line_9_4_05e2d : Inport  Port=2
  State_vq_bus_4_f2dcb : Inport  Port=3
  State_vq_bus_9_57552 : Inport  Port=4
  Add_94035 : Sum
  Constant_-376.991118430775_e6da7 : Constant  Value=-376.991118430775
  Constant_4371.69644539061_2c4ac : Constant  Value=4371.69644539061
  Constant_4371.69644539061_b148a : Constant  Value=4371.69644539061
  Constant_46.8081143789666_d10ec : Constant  Value=46.8081143789666
  Product_63ec8 : Product
  Product_84ab7 : Product
  Product_86c30 : Product
  Product_c1cff : Product
  Subtract_15de9 : Sum  Inputs=+-
  Subtract_30dae : Sum  Inputs=+-
  Blockout_d_iq_line_9_4_dbc5a : Outport
  wires:
  Constant_-376.991118430775_e6da7/1 -> Product_84ab7/1
  Constant_46.8081143789666_d10ec/1 -> Product_86c30/1
  State_id_line_9_4_c69ca/1 -> Product_84ab7/2
  State_iq_line_9_4_05e2d/1 -> Product_86c30/2
  Product_84ab7/1 -> Subtract_15de9/1
  Constant_4371.69644539061_b148a/1 -> Product_63ec8/1
  Product_86c30/1 -> Subtract_15de9/2
  State_vq_bus_4_f2dcb/1 -> Product_63ec8/2
  Subtract_15de9/1 -> Subtract_30dae/1
  Product_63ec8/1 -> Subtract_30dae/2
  Constant_4371.69644539061_2c4ac/1 -> Product_c1cff/1
  Add_94035/1 -> Blockout_d_iq_line_9_4_dbc5a/1
  State_vq_bus_9_57552/1 -> Product_c1cff/2
  Subtract_30dae/1 -> Add_94035/1
  Product_c1cff/1 -> Add_94035/2

== system case9/AC_1/d_iq_load_5_block ==
  note: d_iq_load_5 in case9
      | $1369.24920855552\,\mathrm{vq}_{\mathrm{bus},5}-1271.35173163011\,\mathrm{iq}_{\mathrm{load},5}-376.991118430775\,\mathrm{id}_{\mathrm{load},5}$
      | Automatically generated on 2025-10-31 19:35:38 .
  State_id_load_5_f81f9 : Inport
  State_iq_load_5_ffc98 : Inport  Port=2
  State_vq_bus_5_63e45 : Inport  Port=3
  Add_58200 : Sum
  Constant_-376.991118430775_2f218 : Constant  Value=-376.991118430775
  Constant_1271.35173163011_f87c3 : Constant  Value=1271.35173163011
  Constant_1369.24920855552_4752a : Constant  Value=1369.24920855552
  Product_9e825 : Product
  Product_b583a : Product
  Product_ed628 : Product
  Subtract_5ca1d : Sum  Inputs=+-
  Blockout_d_iq_load_5_51512 : Outport
  wires:
  Constant_-376.991118430775_2f218/1 -> Product_ed628/1
  Product_9e825/1 -> Subtract_5ca1d/2
  State_id_load_5_f81f9/1 -> Product_ed628/2
  Constant_1271.35173163011_f87c3/1 -> Product_9e825/1
  Product_ed628/1 -> Subtract_5ca1d/1
  State_iq_load_5_ffc98/1 -> Product_9e825/2
  Constant_1369.24920855552_4752a/1 -> Product_b583a/1
  State_vq_bus_5_63e45/1 -> Product_b583a/2
  Subtract_5ca1d/1 -> Add_58200/1
  Product_b583a/1 -> Add_58200/2
  Add_58200/1 -> Blockout_d_iq_load_5_51512/1

== system case9/AC_1/d_iq_load_7_block ==
  note: d_iq_load_7 in case9
      | $1430.28886940914\,\mathrm{vq}_{\mathrm{bus},7}-1210.81117316871\,\mathrm{iq}_{\mathrm{load},7}-376.991118430775\,\mathrm{id}_{\mathrm{load},7}$
      | Automatically generated on 2025-10-31 19:35:38 .
  State_id_load_7_4efb5 : Inport
  State_iq_load_7_52d58 : Inport  Port=2
  State_vq_bus_7_4c107 : Inport  Port=3
  Add_f0538 : Sum
  Constant_-376.991118430775_1c537 : Constant  Value=-376.991118430775
  Constant_1210.81117316871_f4ffd : Constant  Value=1210.81117316871
  Constant_1430.28886940914_10292 : Constant  Value=1430.28886940914
  Product_4aa54 : Product
  Product_860f3 : Product
  Product_fb31b : Product
  Subtract_6579a : Sum  Inputs=+-
  Blockout_d_iq_load_7_8aad1 : Outport
  wires:
  Constant_-376.991118430775_1c537/1 -> Product_860f3/1
  Product_fb31b/1 -> Subtract_6579a/2
  State_id_load_7_4efb5/1 -> Product_860f3/2
  Constant_1210.81117316871_f4ffd/1 -> Product_fb31b/1
  Product_860f3/1 -> Subtract_6579a/1
  State_iq_load_7_52d58/1 -> Product_fb31b/2
  Constant_1430.28886940914_10292/1 -> Product_4aa54/1
  State_vq_bus_7_4c107/1 -> Product_4aa54/2
  Subtract_6579a/1 -> Add_f0538/1
  Product_4aa54/1 -> Add_f0538/2
  Add_f0538/1 -> Blockout_d_iq_load_7_8aad1/1

== system case9/AC_1/d_iq_load_9_block ==
  note: d_iq_load_9 in case9
      | $1700.21710984812\,\mathrm{vq}_{\mathrm{bus},9}-1059.45977647\,\mathrm{iq}_{\mathrm{load},9}-376.991118430775\,\mathrm{id}_{\mathrm{load},9}$
      | Automatically generated on 2025-10-31 19:35:39 .
  State_id_load_9_ca328 : Inport
  State_iq_load_9_18565 : Inport  Port=2
  State_vq_bus_9_b75c9 : Inport  Port=3
  Add_2afe8 : Sum
  Constant_-376.991118430775_25dfb : Constant  Value=-376.991118430775
  Constant_1059.45977647_8f20d : Constant  Value=1059.45977647
  Constant_1700.21710984812_bf71d : Constant  Value=1700.21710984812
  Product_49255 : Product
  Product_bd907 : Product
  Product_f35ca : Product
  Subtract_265ab : Sum  Inputs=+-
  Blockout_d_iq_load_9_b92e3 : Outport
  wires:
  Constant_-376.991118430775_25dfb/1 -> Product_f35ca/1
  Product_bd907/1 -> Subtract_265ab/2
  State_id_load_9_ca328/1 -> Product_f35ca/2
  Add_2afe8/1 -> Blockout_d_iq_load_9_b92e3/1
  Constant_1059.45977647_8f20d/1 -> Product_bd907/1
  Product_49255/1 -> Add_2afe8/2
  Product_f35ca/1 -> Subtract_265ab/1
  State_iq_load_9_18565/1 -> Product_bd907/2
  Constant_1700.21710984812_bf71d/1 -> Product_49255/1
  State_vq_bus_9_b75c9/1 -> Product_49255/2
  Subtract_265ab/1 -> Add_2afe8/1

== system case9/AC_1/d_vd_bus_1_block ==
  note: d_vd_bus_1 in case9
      | $37699111.8430775\,\mathrm{id}_{\mathrm{bus},1}+376.991118430775\,\mathrm{vq}_{\mathrm{bus},1}$
      | Automatically generated on 2025-10-31 19:35:33 .
  Alge_id_bus_1_d6354 : Inport
  State_vq_bus_1_f7898 : Inport  Port=2
  Add_fb20c : Sum
  Constant_376.991118430775_a2214 : Constant  Value=376.991118430775
  Constant_37699111.8430775_99d01 : Constant  Value=37699111.8430775
  Product_40e41 : Product
  Product_77053 : Product
  Blockout_d_vd_bus_1_2d89b : Outport
  wires:
  Constant_37699111.8430775_99d01/1 -> Product_77053/1
  Product_40e41/1 -> Add_fb20c/2
  Alge_id_bus_1_d6354/1 -> Product_77053/2
  Constant_376.991118430775_a2214/1 -> Product_40e41/1
  State_vq_bus_1_f7898/1 -> Product_40e41/2
  Add_fb20c/1 -> Blockout_d_vd_bus_1_2d89b/1
  Product_77053/1 -> Add_fb20c/1

== system case9/AC_1/d_vd_bus_2_block ==
  note: d_vd_bus_2 in case9
      | $37699111.8430775\,\mathrm{id}_{\mathrm{bus},2}+376.991118430775\,\mathrm{vq}_{\mathrm{bus},2}$
      | Automatically generated on 2025-10-31 19:35:33 .
  Alge_id_bus_2_03e19 : Inport
  State_vq_bus_2_79979 : Inport  Port=2
  Add_a50b6 : Sum
  Constant_376.991118430775_61ba1 : Constant  Value=376.991118430775
  Constant_37699111.8430775_eb154 : Constant  Value=37699111.8430775
  Product_11bc3 : Product
  Product_d95da : Product
  Blockout_d_vd_bus_2_239dc : Outport
  wires:
  Constant_37699111.8430775_eb154/1 -> Product_11bc3/1
  Product_d95da/1 -> Add_a50b6/2
  Alge_id_bus_2_03e19/1 -> Product_11bc3/2
  Constant_376.991118430775_61ba1/1 -> Product_d95da/1
  Product_11bc3/1 -> Add_a50b6/1
  State_vq_bus_2_79979/1 -> Product_d95da/2
  Add_a50b6/1 -> Blockout_d_vd_bus_2_239dc/1

== system case9/AC_1/d_vd_bus_3_block ==
  note: d_vd_bus_3 in case9
      | $37699111.8430775\,\mathrm{id}_{\mathrm{bus},3}+376.991118430775\,\mathrm{vq}_{\mathrm{bus},3}$
      | Automatically generated on 2025-10-31 19:35:34 .
  Alge_id_bus_3_75936 : Inport
  State_vq_bus_3_e0598 : Inport  Port=2
  Add_28de6 : Sum
  Constant_376.991118430775_4166b : Constant  Value=376.991118430775
  Constant_37699111.8430775_79e01 : Constant  Value=37699111.8430775
  Product_c64f7 : Product
  Product_fb217 : Product
  Blockout_d_vd_bus_3_cd175 : Outport
  wires:
  Constant_37699111.8430775_79e01/1 -> Product_fb217/1
  Product_c64f7/1 -> Add_28de6/2
  Alge_id_bus_3_75936/1 -> Product_fb217/2
  Constant_376.991118430775_4166b/1 -> Product_c64f7/1
  Product_fb217/1 -> Add_28de6/1
  State_vq_bus_3_e0598/1 -> Product_c64f7/2
  Add_28de6/1 -> Blockout_d_vd_bus_3_cd175/1

== system case9/AC_1/d_vd_bus_4_block ==
  note: d_vd_bus_4 in case9
      | $2257.43184689087\,\mathrm{id}_{\mathrm{bus},4}+376.991118430775\,\mathrm{vq}_{\mathrm{bus},4}$
      | Automatically generated on 2025-10-31 19:35:34 .
  Alge_id_bus_4_ba533 : Inport
  State_vq_bus_4_1829b : Inport  Port=2
  Add_af20f : Sum
  Constant_2257.43184689087_6450d : Constant  Value=2257.43184689087
  Constant_376.991118430775_d32c1 : Constant  Value=376.991118430775
  Product_5f240 : Product
  Product_94d15 : Product
  Blockout_d_vd_bus_4_13a25 : Outport
  wires:
  Constant_2257.43184689087_6450d/1 -> Product_5f240/1
  Product_94d15/1 -> Add_af20f/2
  Alge_id_bus_4_ba533/1 -> Product_5f240/2
  Constant_376.991118430775_d32c1/1 -> Product_94d15/1
  Product_5f240/1 -> Add_af20f/1
  State_vq_bus_4_1829b/1 -> Product_94d15/2
  Add_af20f/1 -> Blockout_d_vd_bus_4_13a25/1

== system case9/AC_1/d_vd_bus_5_block ==
  note: d_vd_bus_5 in case9
      | $1461.2058853906\,\mathrm{id}_{\mathrm{bus},5}+376.991118430775\,\mathrm{vq}_{\mathrm{bus},5}$
      | Automatically generated on 2025-10-31 19:35:35 .
  Alge_id_bus_5_0947a : Inport
  State_vq_bus_5_7a578 : Inport  Port=2
  Add_a061a : Sum
  Constant_1461.2058853906_d832d : Constant  Value=1461.2058853906
  Constant_376.991118430775_188e7 : Constant  Value=376.991118430775
  Product_68369 : Product
  Product_8e6b8 : Product
  Blockout_d_vd_bus_5_11407 : Outport
  wires:
  Constant_1461.2058853906_d832d/1 -> Product_68369/1
  Product_8e6b8/1 -> Add_a061a/2
  Alge_id_bus_5_0947a/1 -> Product_68369/2
  Constant_376.991118430775_188e7/1 -> Product_8e6b8/1
  Product_68369/1 -> Add_a061a/1
  State_vq_bus_5_7a578/1 -> Product_8e6b8/2
  Add_a061a/1 -> Blockout_d_vd_bus_5_11407/1

== system case9/AC_1/d_vd_bus_6_block ==
  note: d_vd_bus_6 in case9
      | $1329.77466818616\,\mathrm{id}_{\mathrm{bus},6}+376.991118430775\,\mathrm{vq}_{\mathrm{bus},6}$
      | Automatically generated on 2025-10-31 19:35:35 .
  Alge_id_bus_6_03468 : Inport
  State_vq_bus_6_65470 : Inport  Port=2
  Add_d3b4a : Sum
  Constant_1329.77466818616_1621f : Constant  Value=1329.77466818616
  Constant_376.991118430775_0b28d : Constant  Value=376.991118430775
  Product_26d7a : Product
  Product_e2a74 : Product
  Blockout_d_vd_bus_6_2017b : Outport
  wires:
  Constant_1329.77466818616_1621f/1 -> Product_26d7a/1
  Product_e2a74/1 -> Add_d3b4a/2
  Alge_id_bus_6_03468/1 -> Product_26d7a/2
  Constant_376.991118430775_0b28d/1 -> Product_e2a74/1
  Product_26d7a/1 -> Add_d3b4a/1
  State_vq_bus_6_65470/1 -> Product_e2a74/2
  Add_d3b4a/1 -> Blockout_d_vd_bus_6_2017b/1

== system case9/AC_1/d_vd_bus_7_block ==
  note: d_vd_bus_7 in case9
      | $2106.09563369148\,\mathrm{id}_{\mathrm{bus},7}+376.991118430775\,\mathrm{vq}_{\mathrm{bus},7}$
      | Automatically generated on 2025-10-31 19:35:36 .
  Alge_id_bus_7_4fc23 : Inport
  State_vq_bus_7_8c2e9 : Inport  Port=2
  Add_42fa3 : Sum
  Constant_2106.09563369148_04e9b : Constant  Value=2106.09563369148
  Constant_376.991118430775_92bbe : Constant  Value=376.991118430775
  Product_54305 : Product
  Product_87a75 : Product
  Blockout_d_vd_bus_7_67ab2 : Outport
  wires:
  Constant_2106.09563369148_04e9b/1 -> Product_87a75/1
  Product_54305/1 -> Add_42fa3/2
  Alge_id_bus_7_4fc23/1 -> Product_87a75/2
  Constant_376.991118430775_92bbe/1 -> Product_54305/1
  Product_87a75/1 -> Add_42fa3/1
  State_vq_bus_7_8c2e9/1 -> Product_54305/2
  Add_42fa3/1 -> Blockout_d_vd_bus_7_67ab2/1

== system case9/AC_1/d_vd_bus_8_block ==
  note: d_vd_bus_8 in case9
      | $1657.10381727813\,\mathrm{id}_{\mathrm{bus},8}+376.991118430775\,\mathrm{vq}_{\mathrm{bus},8}$
      | Automatically generated on 2025-10-31 19:35:36 .
  Alge_id_bus_8_b8a05 : Inport
  State_vq_bus_8_fa58b : Inport  Port=2
  Add_25f48 : Sum
  Constant_1657.10381727813_c6477 : Constant  Value=1657.10381727813
  Constant_376.991118430775_2e96a : Constant  Value=376.991118430775
  Product_815e8 : Product
  Product_abbb7 : Product
  Blockout_d_vd_bus_8_4b188 : Outport
  wires:
  Constant_1657.10381727813_c6477/1 -> Product_815e8/1
  Product_abbb7/1 -> Add_25f48/2
  Alge_id_bus_8_b8a05/1 -> Product_815e8/2
  Constant_376.991118430775_2e96a/1 -> Product_abbb7/1
  Product_815e8/1 -> Add_25f48/1
  State_vq_bus_8_fa58b/1 -> Product_abbb7/2
  Add_25f48/1 -> Blockout_d_vd_bus_8_4b188/1

== system case9/AC_1/d_vd_bus_9_block ==
  note: d_vd_bus_9 in case9
      | $1564.27849971276\,\mathrm{id}_{\mathrm{bus},9}+376.991118430775\,\mathrm{vq}_{\mathrm{bus},9}$
      | Automatically generated on 2025-10-31 19:35:37 .
  Alge_id_bus_9_dcda6 : Inport
  State_vq_bus_9_f0504 : Inport  Port=2
  Add_0ca8a : Sum
  Constant_1564.27849971276_8a32b : Constant  Value=1564.27849971276
  Constant_376.991118430775_d0374 : Constant  Value=376.991118430775
  Product_04e37 : Product
  Product_5a3d6 : Product
  Blockout_d_vd_bus_9_26b07 : Outport
  wires:
  Constant_1564.27849971276_8a32b/1 -> Product_5a3d6/1
  Product_04e37/1 -> Add_0ca8a/2
  Alge_id_bus_9_dcda6/1 -> Product_5a3d6/2
  Constant_376.991118430775_d0374/1 -> Product_04e37/1
  Product_5a3d6/1 -> Add_0ca8a/1
  State_vq_bus_9_f0504/1 -> Product_04e37/2
  Add_0ca8a/1 -> Blockout_d_vd_bus_9_26b07/1

== system case9/AC_1/d_vq_bus_1_block ==
  note: d_vq_bus_1 in case9
      | $37699111.8430775\,\mathrm{iq}_{\mathrm{bus},1}-376.991118430775\,\mathrm{vd}_{\mathrm{bus},1}$
      | Automatically generated on 2025-10-31 19:35:33 .
  Alge_iq_bus_1_08517 : Inport
  State_vd_bus_1_cc6f2 : Inport  Port=2
  Constant_376.991118430775_1e099 : Constant  Value=376.991118430775
  Constant_37699111.8430775_4f84c : Constant  Value=37699111.8430775
  Product_5383c : Product
  Product_ab7b3 : Product
  Subtract_a6450 : Sum  Inputs=+-
  Blockout_d_vq_bus_1_ac2d6 : Outport
  wires:
  Constant_37699111.8430775_4f84c/1 -> Product_ab7b3/1
  Constant_376.991118430775_1e099/1 -> Product_5383c/1
  Alge_iq_bus_1_08517/1 -> Product_ab7b3/2
  State_vd_bus_1_cc6f2/1 -> Product_5383c/2
  Product_ab7b3/1 -> Subtract_a6450/1
  Product_5383c/1 -> Subtract_a6450/2
  Subtract_a6450/1 -> Blockout_d_vq_bus_1_ac2d6/1
